simulink model "Modelo_Red_Mitigación_final"  (R2019b)
settings: Solver=VariableStepAuto  StartTime=0.0  StopTime=2.5  RelTol=1e-3
InitFcn:
  | Ts=20e-6;
undefined symbols (not defined in the file): D1, Delta, Ion, Lithium
libraries: powerlib x371, powerlib_meascontrol x286, simulink x50, simulink_extras x20, electricdrivelib x16
(part 8 of 11)

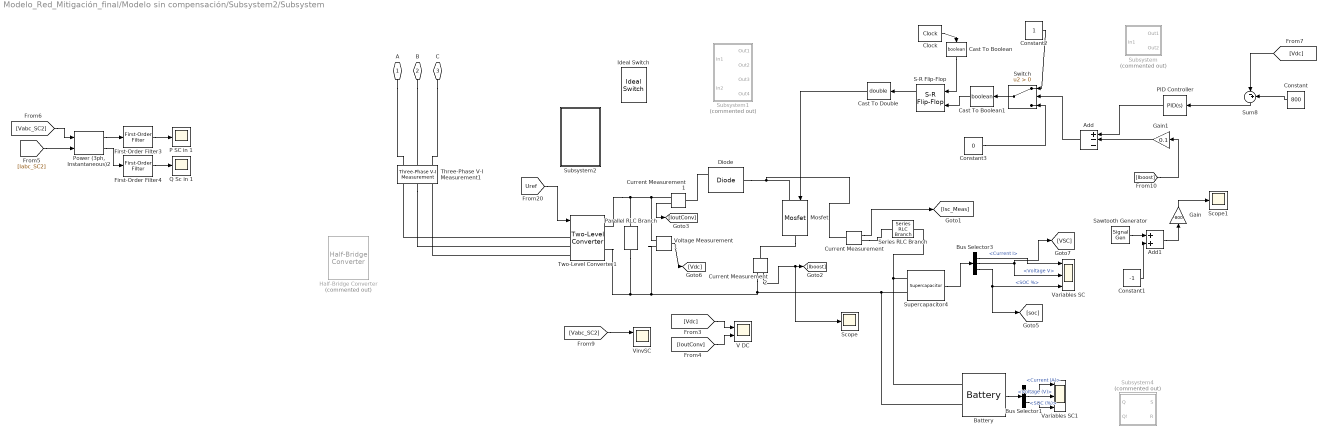
== system Modelo_Red_Mitigación_final/Modelo sin compensación/Subsystem2/Subsystem ==
  Add : Sum  Inputs=+--
  Add1 : Sum
  Battery : electricdrivelib/Extra Sources/Battery  BatType=Lithium-Ion  ShowTempParam=off  ThermalPreset=no  ShowAgeParam=off  NomV=500  NomQ=500  SOC=100  Batt_Tr=30  PresetModel=on  MaxQ=500  MinV=375  FullV=581.9936  Dis_rate=217.3913  R=0.01  Normal_OP=452.1739  expZone="[540.1929      24.56522]"  current=[6.5 13 32.5]  Units=Time  Tci=20  NomT=20  T2=-30  MaxQ2=4.8  FullV2=7.1  Normal_OP2=5.655  expZone2="[6.58           1]"  Rca=0.6  ti=2000  Dp=0  Neq0=0  Tsim=1e6  Ta1=25  Qeol=5.4*0.9  Reol=0.013333*1.2  Char_age=[2.3478, 3]  Dis_age=[2.3478, 10]  N1=1500  N2=10500  N3=1000  N4=1400  Ta2=45  N5=950
      settings: SourceProductName=Simscape Electrical
  Bus Selector1 : BusSelector  OutputSignals=Current (A),Voltage (V),SOC (%)
  Bus Selector3 : BusSelector  OutputSignals=Current I,Voltage V,SOC %
  Cast To Boolean : DataTypeConversion  OutDataTypeStr=boolean
  Cast To Boolean1 : DataTypeConversion  OutDataTypeStr=boolean
  Cast To Double : DataTypeConversion  OutDataTypeStr=double
  Clock : simulink_extras/Flip Flops/Clock  period=1/10e3
  Constant : Constant  Value=800
  Constant1 : Constant  Value=-1
  Constant2 : Constant
  Constant3 : Constant  Value=0
  Current Measurement : powerlib/Measurements/Current Measurement  PhasorSimulation=off  OutputType=Complex  PSBequivalent=0
      settings: SourceProductName=Simscape Electrical
  Current Measurement1 : powerlib/Measurements/Current Measurement  PhasorSimulation=off  OutputType=Complex  PSBequivalent=0
      settings: SourceProductName=Simscape Electrical
  Current Measurement2 : powerlib/Measurements/Current Measurement  PhasorSimulation=off  OutputType=Complex  PSBequivalent=0
      settings: SourceProductName=Simscape Electrical
  Diode : powerlib/Power Electronics/Diode  Ron=0.001  Lon=0  Vf=0.8  IC=0  UseSnubber=0  Rs=500  Cs=250e-9  Measurements=on
      settings: SourceProductName=Simscape Electrical
  First-Order Filter3 : powerlib_meascontrol/Filters/First-Order Filter  FilterType=Lowpass  Tc=10e-3  Ts=0  Initialize=on  Vac_Init=[0, 0, 60]  Vdc_Init=0  PlotResponse=off  FreqRange="[0,  200,  1]"
      settings: SourceProductName=Simscape Electrical
  First-Order Filter4 : powerlib_meascontrol/Filters/First-Order Filter  FilterType=Lowpass  Tc=10e-3  Ts=0  Initialize=on  Vac_Init=[0, 0, 60]  Vdc_Init=0  PlotResponse=off  FreqRange="[0,  200,  1]"
      settings: SourceProductName=Simscape Electrical
  Gain : Gain  Gain=-800
  Gain1 : Gain  Gain=0.1
  Half-Bridge Converter : powerlib/Power Electronics/Half-Bridge Converter  Commented=on  ModelType=Switching devices  Ron=1e-3  Rs=1e6  Cs=inf  Vforward=[0,0]  Ron_Diode=1e-3  Rs_Diode=1e6  Cs_Diode=inf  Vf_Diode=1e-3  Rs_CurrentSource=inf
      settings: SourceProductName=Simscape Electrical  SourceProductBaseCode=PS
  Ideal Switch : powerlib/Power Electronics/Ideal Switch  Ron=1e-3  Lon=0  IC=1  Rs=1e5  Cs=inf  Measurements=on
      settings: SourceProductName=Simscape Electrical
  Mosfet : powerlib/Power Electronics/Mosfet  Ron=0.1  Lon=0  Rd=0.01  Vfd=0  IC=0  Rs=1e5  Cs=inf  Measurements=off
      settings: SourceProductName=Simscape Electrical
  P SC in 1 : Scope
  PID Controller : simulink/Continuous/PID Controller  Controller=PID  Form=Parallel  TimeDomain=Continuous-time  SampleTime=-1  IntegratorMethod=Forward Euler  FilterMethod=Forward Euler  ControllerParametersSource=internal  P=40  I=10  D=0  UseFilter=on  N=100  TunerSelectOption=Transfer Function Based (PID Tuner App)  InitialConditionSource=internal  InitialConditionForIntegrator=0  InitialConditionForFilter=0  DifferentiatorICPrevScaledInput=0  ExternalReset=none  TrackingMode=off  Kt=1  LimitOutput=off  UpperSaturationLimit=inf  LowerSaturationLimit=-inf  LinearizeAsGain=on  AntiWindupMode=none  Kb=1  POutMin=[]  POutMax=[]  IOutMin=[]  IOutMax=[]  DOutMin=[]  DOutMax=[]  NOutMin=[]  NOutMax=[]  SumOutMin=[]  SumOutMax=[]  SaturationOutMin=[]  SaturationOutMax=[]  PParamMin=[]  PParamMax=[]  IParamMin=[]  IParamMax=[]  DParamMin=[]  DParamMax=[]  NParamMin=[]  NParamMax=[]  KbParamMin=[]  KbParamMax=[]  KtParamMin=[]  KtParamMax=[]  KbOutMin=[]  KbOutMax=[]  KtOutMin=[]  KtOutMax=[]  IntegratorOutMin=[]  IntegratorOutMax=[]  FilterOutMin=[]  FilterOutMax=[]  SumI1OutMin=[]  SumI1OutMax=[]  SumI2OutMin=[]  SumI2OutMax=[]  SumI3OutMin=[]  SumI3OutMax=[]  SumI4OutMin=[]  SumI4OutMax=[]  SumDOutMin=[]  SumDOutMax=[]  DifferentiatorOutMin=[]  DifferentiatorOutMax=[]  FilterDiffOutCoefMin=[]  FilterDiffOutCoefMax=[]  ReciprocalOutMin=[]  ReciprocalOutMax=[]  SumDenOutMin=[]  SumDenOutMax=[]  SumNumOutMin=[]  SumNumOutMax=[]  DivideOutMin=[]  DivideOutMax=[]  IntegratorContinuousStateAttributes=''  IntegratorStateMustResolveToSignalObject=off  IntegratorRTWStateStorageClass=Auto  FilterContinuousStateAttributes=''  FilterStateMustResolveToSignalObject=off  FilterRTWStateStorageClass=Auto  ParallelPVariant=InternalParameters  IdealPVariant=Disabled  IVariant=InternalParameters  DVariant=InternalParameters  IntegratorVariant=Continuous  SatVariant=Disabled  AWVariant=Passthrough  PCopyVariant=Disabled  TRVariant=Disabled  FdbkBlocksVariant=Forward  IdealPFdbkVariant=Disabled  SatFdbkVariant=Disabled  DerivativeFilterVariant=ContFilter  NVariant=InternalParameters  NCopyVariant=Disabled  FilterICVariant=InternalICsFilter  IntegratorICVariant=InternalICs  ExternalResetVariant=Disabled  TRSumVariant=Passthrough  SumFdbkVariant=Disabled  SumVariant=Sum_PID
  Parallel RLC Branch : powerlib/Elements/Parallel RLC Branch  LConnTagsString=a  RConnTagsString=__new0  BranchType=C  Resistance=0.01  Inductance=1e-3  SetiL0=off  InitialCurrent=0  Capacitance=6600e-6  Setx0=off  InitialVoltage=800  Measurements=None
      settings: SourceProductName=Simscape Electrical
  "Power (3ph, Instantaneous)2" : powerlib_meascontrol/Measurements/Power (3ph, Instantaneous)
      settings: SourceProductName=Simscape Electrical
  Q Sc in 1 : Scope
  S-R Flip-Flop : simulink_extras/Flip Flops/S-R Flip-Flop  initial_condition=1
  Sawtooth Generator : SignalGenerator  WaveForm=sawtooth  Frequency=10e3
  Scope : Scope
  Scope1 : Scope
  Series RLC Branch : powerlib/Elements/Series RLC Branch  LConnTagsString=__new0  RConnTagsString=__new0  BranchType=L  Resistance=65e-3  Inductance=1e-3  SetiL0=off  InitialCurrent=0  Capacitance=1e-6  Setx0=off  InitialVoltage=0  Measurements=None
      settings: SourceProductName=Simscape Electrical
  Subsystem : Subsystem  Commented=on
  Subsystem1 : Subsystem  Commented=on
  Subsystem2 : Subsystem
  Subsystem4 : Subsystem  Commented=on
  Sum8 : Sum  Inputs=|-+
  Supercapacitor4 : electricdrivelib/Extra Sources/Supercapacitor  C=18  Rdc=7e-3  Voltage=500  Ns=1  Np=1  Vinit=500  Temp=25  PresetModel=on  EstParam=off  Nc=1  r=1e-9  epsilon=6.0208e-10  Ich=10  Vstern="[0.161  2.7  7.8]"  Self_dis=off  Ioc=10  Vself="[48  47.8  47.06  44.65]"  demandeplot=off  I="[10  20 100  500]"  Units=sec  Vmax=0  If=0  deltaV=0  alpha=0  sec=0
      settings: SourceProductName=Simscape Electrical  SourceProductBaseCode=PS
  Switch : Switch  Criteria=u2 > Threshold
  Three-Phase V-I Measurement1 : powerlib/Measurements/Three-Phase V-I Measurement  VoltageMeasurement=phase-to-phase  SetLabelV=on  LabelV=Vabc_SC2  Vpu=off  VpuLL=off  CurrentMeasurement=yes  SetLabelI=on  LabelI=Iabc_SC2  Ipu=off  Pbase=100e6  Vbase=500e3  OutputType=Complex  PhasorSimulation=off  PSBequivalent=0
      settings: SourceProductName=Simscape Electrical
  Two-Level Converter1 : powerlib/Power Electronics/Two-Level Converter  ModelType=Average model (Uref-controlled)  Ron=1e-3  Rs=1e6  Cs=inf  Vforward=[0,0]  Ron_Diode=1e-3  Rs_Diode=1e6  Cs_Diode=inf  Vf_Diode=1e-3  Rs_CurrentSource=inf
      settings: SourceProductName=Simscape Electrical  SourceProductBaseCode=PS
  V DC : Scope  NumInputPorts=2
  Variables SC : Scope  NumInputPorts=3
  Variables SC1 : Scope  NumInputPorts=3
  VinvSC : Scope  NumInputPorts=2
  Voltage Measurement1 : powerlib/Measurements/Voltage Measurement  PhasorSimulation=off  OutputType=Complex  PSBequivalent=0
      settings: SourceProductName=Simscape Electrical
  A : PMIOPort  Side=Left
  B : PMIOPort  Port=2  Side=Left
  C : PMIOPort  Port=3  Side=Left
  wires:
  Current Measurement/1 -> [Isc_Meas]
  Bus Selector3/2 -> Variables SC/2, [VSC]  "<Voltage V>"
  Bus Selector3/3 -> [soc], Variables SC/3  "<SOC %>"
  Bus Selector3/1 -> Variables SC/1  "<Current I>"
  "Power (3ph, Instantaneous)2"/2 -> First-Order Filter4/1
  [Iabc_SC2] -> "Power (3ph, Instantaneous)2"/2
  First-Order Filter3/1 -> P SC in 1/1
  [Vabc_SC2] -> "Power (3ph, Instantaneous)2"/1
  First-Order Filter4/1 -> Q Sc in 1/1
  "Power (3ph, Instantaneous)2"/1 -> First-Order Filter3/1
  [Vabc_SC2] -> VinvSC/1
  Voltage Measurement1/1 -> [Vdc]
  [Uref] -> Two-Level Converter1/1
  Current Measurement1/1 -> [IoutConv]
  [Vdc] -> V DC/1
  [IoutConv] -> V DC/2
  Supercapacitor4/1 -> Bus Selector3/1
  Current Measurement2/1 -> Scope/1, [Iboost]
  [Iboost] -> Gain1/1
  Constant/1 -> Sum8/2
  [Vdc] -> Sum8/1
  Cast To Boolean1/1 -> S-R Flip-Flop/2
  Cast To Double/1 -> Mosfet/1
  Clock/1 -> Cast To Boolean/1
  Add/1 -> Switch/2
  Cast To Boolean/1 -> S-R Flip-Flop/1
  S-R Flip-Flop/1 -> Cast To Double/1
  Constant3/1 -> Switch/3
  Switch/1 -> Cast To Boolean1/1
  Constant2/1 -> Switch/1
  Sum8/1 -> PID Controller/1
  Bus Selector1/2 -> Variables SC1/2  "<Voltage (V)>"
  Battery/1 -> Bus Selector1/1
  Bus Selector1/3 -> Variables SC1/3  "<SOC (%)>"
  Bus Selector1/1 -> Variables SC1/1  "<Current (A)>"
  Gain1/1 -> Add/2
  PID Controller/1 -> Add/1
  Sawtooth Generator/1 -> Add1/1
  Add1/1 -> Gain/1
  Constant1/1 -> Add1/2
  Gain/1 -> Scope1/1
  connections:
  Current Measurement/RConn1 -- Series RLC Branch/LConn1
  Voltage Measurement1/LConn2 -- Battery/LConn2 -- Supercapacitor4/LConn2 -- Current Measurement2/RConn1 -- Two-Level Converter1/RConn2 -- Parallel RLC Branch/RConn1
  B/RConn1 -- Three-Phase V-I Measurement1/LConn2
  C/RConn1 -- Three-Phase V-I Measurement1/LConn3
  A/RConn1 -- Three-Phase V-I Measurement1/LConn1
  Parallel RLC Branch/LConn1 -- Two-Level Converter1/RConn1 -- Current Measurement1/RConn1 -- Voltage Measurement1/LConn1
  Diode/LConn1 -- Mosfet/LConn1 -- Current Measurement/LConn1
  Two-Level Converter1/LConn1 -- Three-Phase V-I Measurement1/RConn1
  Three-Phase V-I Measurement1/RConn2 -- Two-Level Converter1/LConn2
  Two-Level Converter1/LConn3 -- Three-Phase V-I Measurement1/RConn3
  Mosfet/RConn1 -- Current Measurement2/LConn1
  Diode/RConn1 -- Current Measurement1/LConn1
  Supercapacitor4/LConn1 -- Battery/LConn1 -- Series RLC Branch/RConn1

== system Modelo_Red_Mitigación_final/Modelo SC pasivo/Subsystem2/Subsystem/Subsystem ==
  In1 : Inport
  Cast To Boolean : DataTypeConversion  OutDataTypeStr=boolean
  Cast To Boolean1 : DataTypeConversion  OutDataTypeStr=boolean
  Cast To Double : DataTypeConversion  OutDataTypeStr=double
  Clock : simulink_extras/Flip Flops/Clock  period=1/10e3
  Constant1 : Constant  Value=0
  Constant2 : Constant
  Constant3 : Constant  Value=0
  Mux : Mux  Inputs=2
  S-R Flip-Flop : simulink_extras/Flip Flops/S-R Flip-Flop  initial_condition=1
  Switch : Switch  Criteria=u2 > Threshold
  Out1 : Outport
  Out2 : Outport  Port=2
  wires:
  S-R Flip-Flop/1 -> Cast To Double/1
  Constant2/1 -> Switch/1
  Cast To Double/1 -> Mux/2
  Cast To Boolean/1 -> S-R Flip-Flop/1
  Constant1/1 -> Mux/1
  Constant3/1 -> Switch/3
  Switch/1 -> Cast To Boolean1/1
  Cast To Boolean1/1 -> S-R Flip-Flop/2
  Mux/1 -> Out1/1
  Clock/1 -> Cast To Boolean/1
  In1/1 -> Switch/2
  S-R Flip-Flop/2 -> Out2/1

== system Modelo_Red_Mitigación_final/Modelo SC pasivo/Subsystem2/Subsystem/Subsystem1 ==
  In1 : Inport
  In2 : Inport  Port=2
  Constant2 : Constant
  Constant3 : Constant  Value=100
  Constant4 : Constant
  Demux1 : Demux  Outputs=3
  First-Order Filter : powerlib_meascontrol/Filters/First-Order Filter  FilterType=Lowpass  Tc=10e-3  Ts=0  Initialize=on  Vac_Init=[0, 0, 60]  Vdc_Init=0  PlotResponse=off  FreqRange="[0,  200,  1]"
      settings: SourceProductName=Simscape Electrical
  Gain : Gain  Gain=1/1200
  Gain1 : Gain  Gain=pi/180
  Gain2 : Gain  Gain=1/254
  Gain3 : Gain  Gain=1/30e3
  Isc : Scope
  MATLAB Function : MATLAB Function  TreatAsAtomicUnit=on
  Memory1 : Memory
  Memory2 : Memory
  Mux2 : Mux  Inputs=3
  Mux3 : Mux  Inputs=3
  PID Controller1 : simulink/Continuous/PID Controller  Controller=PID  Form=Parallel  TimeDomain=Discrete-time  SampleTime=-1  IntegratorMethod=Forward Euler  FilterMethod=Forward Euler  ControllerParametersSource=internal  P=0.4  I=1  D=0  UseFilter=off  N=100  TunerSelectOption=Transfer Function Based (PID Tuner App)  InitialConditionSource=internal  InitialConditionForIntegrator=0.5  InitialConditionForFilter=0.5  DifferentiatorICPrevScaledInput=0  ExternalReset=none  TrackingMode=off  Kt=1  LimitOutput=off  UpperSaturationLimit=inf  LowerSaturationLimit=-inf  LinearizeAsGain=on  AntiWindupMode=none  Kb=1  POutMin=[]  POutMax=[]  IOutMin=[]  IOutMax=[]  DOutMin=[]  DOutMax=[]  NOutMin=[]  NOutMax=[]  SumOutMin=[]  SumOutMax=[]  SaturationOutMin=[]  SaturationOutMax=[]  PParamMin=[]  PParamMax=[]  IParamMin=[]  IParamMax=[]  DParamMin=[]  DParamMax=[]  NParamMin=[]  NParamMax=[]  KbParamMin=[]  KbParamMax=[]  KtParamMin=[]  KtParamMax=[]  KbOutMin=[]  KbOutMax=[]  KtOutMin=[]  KtOutMax=[]  IntegratorOutMin=[]  IntegratorOutMax=[]  FilterOutMin=[]  FilterOutMax=[]  SumI1OutMin=[]  SumI1OutMax=[]  SumI2OutMin=[]  SumI2OutMax=[]  SumI3OutMin=[]  SumI3OutMax=[]  SumI4OutMin=[]  SumI4OutMax=[]  SumDOutMin=[]  SumDOutMax=[]  DifferentiatorOutMin=[]  DifferentiatorOutMax=[]  FilterDiffOutCoefMin=[]  FilterDiffOutCoefMax=[]  ReciprocalOutMin=[]  ReciprocalOutMax=[]  SumDenOutMin=[]  SumDenOutMax=[]  SumNumOutMin=[]  SumNumOutMax=[]  DivideOutMin=[]  DivideOutMax=[]  IntegratorContinuousStateAttributes=''  IntegratorStateMustResolveToSignalObject=off  IntegratorRTWStateStorageClass=Auto  FilterContinuousStateAttributes=''  FilterStateMustResolveToSignalObject=off  FilterRTWStateStorageClass=Auto  ParallelPVariant=InternalParameters  IdealPVariant=Disabled  IVariant=InternalParameters  DVariant=InternalParameters  IntegratorVariant=Discrete  SatVariant=Disabled  AWVariant=Passthrough  PCopyVariant=Disabled  TRVariant=Disabled  FdbkBlocksVariant=Forward  IdealPFdbkVariant=Disabled  SatFdbkVariant=Disabled  DerivativeFilterVariant=Differentiator  NVariant=Passthrough  NCopyVariant=Disabled_SignalSpec  FilterICVariant=InternalICsDifferentiator  IntegratorICVariant=InternalICs  ExternalResetVariant=Disabled  TRSumVariant=Passthrough  SumFdbkVariant=Disabled  SumVariant=Sum_PID
  PID Controller4 : simulink/Continuous/PID Controller  Controller=PID  Form=Parallel  TimeDomain=Discrete-time  SampleTime=-1  IntegratorMethod=Forward Euler  FilterMethod=Forward Euler  ControllerParametersSource=internal  P=0.001  I=0.06  D=0  UseFilter=off  N=100  TunerSelectOption=Transfer Function Based (PID Tuner App)  InitialConditionSource=internal  InitialConditionForIntegrator=0.5  InitialConditionForFilter=0.5  DifferentiatorICPrevScaledInput=0  ExternalReset=none  TrackingMode=off  Kt=1  LimitOutput=off  UpperSaturationLimit=inf  LowerSaturationLimit=-inf  LinearizeAsGain=on  AntiWindupMode=none  Kb=1  POutMin=[]  POutMax=[]  IOutMin=[]  IOutMax=[]  DOutMin=[]  DOutMax=[]  NOutMin=[]  NOutMax=[]  SumOutMin=[]  SumOutMax=[]  SaturationOutMin=[]  SaturationOutMax=[]  PParamMin=[]  PParamMax=[]  IParamMin=[]  IParamMax=[]  DParamMin=[]  DParamMax=[]  NParamMin=[]  NParamMax=[]  KbParamMin=[]  KbParamMax=[]  KtParamMin=[]  KtParamMax=[]  KbOutMin=[]  KbOutMax=[]  KtOutMin=[]  KtOutMax=[]  IntegratorOutMin=[]  IntegratorOutMax=[]  FilterOutMin=[]  FilterOutMax=[]  SumI1OutMin=[]  SumI1OutMax=[]  SumI2OutMin=[]  SumI2OutMax=[]  SumI3OutMin=[]  SumI3OutMax=[]  SumI4OutMin=[]  SumI4OutMax=[]  SumDOutMin=[]  SumDOutMax=[]  DifferentiatorOutMin=[]  DifferentiatorOutMax=[]  FilterDiffOutCoefMin=[]  FilterDiffOutCoefMax=[]  ReciprocalOutMin=[]  ReciprocalOutMax=[]  SumDenOutMin=[]  SumDenOutMax=[]  SumNumOutMin=[]  SumNumOutMax=[]  DivideOutMin=[]  DivideOutMax=[]  IntegratorContinuousStateAttributes=''  IntegratorStateMustResolveToSignalObject=off  IntegratorRTWStateStorageClass=Auto  FilterContinuousStateAttributes=''  FilterStateMustResolveToSignalObject=off  FilterRTWStateStorageClass=Auto  ParallelPVariant=InternalParameters  IdealPVariant=Disabled  IVariant=InternalParameters  DVariant=InternalParameters  IntegratorVariant=Discrete  SatVariant=Disabled  AWVariant=Passthrough  PCopyVariant=Disabled  TRVariant=Disabled  FdbkBlocksVariant=Forward  IdealPFdbkVariant=Disabled  SatFdbkVariant=Disabled  DerivativeFilterVariant=Differentiator  NVariant=Passthrough  NCopyVariant=Disabled_SignalSpec  FilterICVariant=InternalICsDifferentiator  IntegratorICVariant=InternalICs  ExternalResetVariant=Disabled  TRSumVariant=Passthrough  SumFdbkVariant=Disabled  SumVariant=Sum_PID
  PLL (3ph)1 : powerlib_meascontrol/PLL/PLL (3ph)  Fmin=45  Par_Init=[0, 60]  ParK=[180, 3200, 1]  TcD=1e-4  MaxRateChangeFreq=12  FilterCutOffFreq=25  Ts=0  AGC=on
      settings: SourceProductName=Simscape Electrical
  "Power (3ph, Instantaneous)" : powerlib_meascontrol/Measurements/Power (3ph, Instantaneous)
      settings: SourceProductName=Simscape Electrical
  Product : Product
  Product1 : Product
  RMS16 : powerlib_meascontrol/Measurements/RMS  TrueRMS=on  Freq=60  RMSInit=19.9e3  Ts=0
      settings: SourceProductName=Simscape Electrical
  Sin : Trigonometry
  Sum1 : Sum  Inputs=|-+
  Sum4 : Sum  Inputs=+-|
  Sum5 : Sum  Inputs=-+|
  Switch2 : Switch  Criteria=u2 > Threshold  Threshold=0.9
  Tensión bus DC1 : Scope
  Transport Delay : TransportDelay  DelayTime=11.06e-3
  Transport Delay1 : TransportDelay  DelayTime=5.53e-3
  Transport Delay2 : TransportDelay  DelayTime=11.06e-3
  Transport Delay3 : TransportDelay  DelayTime=5.53e-3
  "Uccm " : Scope
  "Uvcm " : Scope
  Out1 : Outport
  Out2 : Outport  Port=2
  Out3 : Outport  Port=3
  Out4 : Outport  Port=4
  wires:
  Gain2/1 -> MATLAB Function/1(u), Switch2/2
  Product1/1 -> Mux3/1, Transport Delay2/1, Transport Delay3/1
  Sin/1 -> [Vabc_sync], Product/1
  [VCli1BT] -> "Power (3ph, Instantaneous)"/1  "V_C2"
  Transport Delay/1 -> Mux2/3
  In2/1 -> [VoutConv]
  Sum5/1 -> Sin/1
  PLL (3ph)1/1 -> Out4/1
  Mux2/1 -> Switch2/1, "Uvcm "/1
  "Power (3ph, Instantaneous)"/1 -> First-Order Filter/1
  Gain/1 -> PID Controller1/1
  Transport Delay2/1 -> Mux3/3
  [soc] -> MATLAB Function/2(soc)
  Product/1 -> Mux2/1, Transport Delay1/1, Transport Delay/1
  Constant4/1 -> Product/2
  PLL (3ph)1/2 -> Sum5/2
  Mux3/1 -> Switch2/3, "Uccm "/1
  [Vabc_sync] -> Product1/1
  [VCli1BT] -> Memory2/1
  Constant2/1 -> Product1/2
  First-Order Filter/1 -> Gain3/1
  MATLAB Function/1(y) -> [Isc_Ref], Isc/1
  Transport Delay1/1 -> Mux2/2
  RMS16/1 -> Gain2/1
  Transport Delay3/1 -> Mux3/2
  "Power (3ph, Instantaneous)"/2 -> Out3/1
  PID Controller4/1 -> Gain1/1
  Memory2/1 -> PLL (3ph)1/1
  Gain3/1 -> Sum4/2
  Demux1/1 -> RMS16/1
  Constant3/1 -> Sum1/2
  PID Controller1/1 -> Tensión bus DC1/1, Sum4/1
  Demux1/3 -> Out2/1
  Gain1/1 -> Sum5/1
  [VCli1BT_1] -> Demux1/1
  In1/1 -> Sum1/1
  Memory1/1 -> PID Controller4/1
  Sum4/1 -> Memory1/1
  Demux1/2 -> Out1/1
  Switch2/1 -> [Uref]
  [ICli1BT] -> "Power (3ph, Instantaneous)"/2  "I_SC Red"
  Sum1/1 -> Gain/1

== system Modelo_Red_Mitigación_final/Modelo SC pasivo/Subsystem2/Subsystem/Subsystem2 ==
  Add : Sum  Inputs=-+
  Constant : Constant  Value=0.95
  Constant1 : Constant  Value=0
  Discrete PID Controller : simulink/Continuous/PID Controller  Controller=PID  Form=Parallel  TimeDomain=Discrete-time  SampleTime=-1  IntegratorMethod=Forward Euler  FilterMethod=Forward Euler  ControllerParametersSource=internal  P=20  I=2  D=0  UseFilter=off  N=100  TunerSelectOption=Transfer Function Based (PID Tuner App)  InitialConditionSource=internal  InitialConditionForIntegrator=0  InitialConditionForFilter=0  DifferentiatorICPrevScaledInput=0  ExternalReset=none  TrackingMode=off  Kt=1  LimitOutput=off  UpperSaturationLimit=inf  LowerSaturationLimit=-inf  LinearizeAsGain=off  AntiWindupMode=none  Kb=1  POutMin=[]  POutMax=[]  IOutMin=[]  IOutMax=[]  DOutMin=[]  DOutMax=[]  NOutMin=[]  NOutMax=[]  SumOutMin=[]  SumOutMax=[]  SaturationOutMin=[]  SaturationOutMax=[]  PParamMin=[]  PParamMax=[]  IParamMin=[]  IParamMax=[]  DParamMin=[]  DParamMax=[]  NParamMin=[]  NParamMax=[]  KbParamMin=[]  KbParamMax=[]  KtParamMin=[]  KtParamMax=[]  KbOutMin=[]  KbOutMax=[]  KtOutMin=[]  KtOutMax=[]  IntegratorOutMin=[]  IntegratorOutMax=[]  FilterOutMin=[]  FilterOutMax=[]  SumI1OutMin=[]  SumI1OutMax=[]  SumI2OutMin=[]  SumI2OutMax=[]  SumI3OutMin=[]  SumI3OutMax=[]  SumI4OutMin=[]  SumI4OutMax=[]  SumDOutMin=[]  SumDOutMax=[]  DifferentiatorOutMin=[]  DifferentiatorOutMax=[]  FilterDiffOutCoefMin=[]  FilterDiffOutCoefMax=[]  ReciprocalOutMin=[]  ReciprocalOutMax=[]  SumDenOutMin=[]  SumDenOutMax=[]  SumNumOutMin=[]  SumNumOutMax=[]  DivideOutMin=[]  DivideOutMax=[]  IntegratorContinuousStateAttributes=''  IntegratorStateMustResolveToSignalObject=off  IntegratorRTWStateStorageClass=Auto  FilterContinuousStateAttributes=''  FilterStateMustResolveToSignalObject=off  FilterRTWStateStorageClass=Auto  ParallelPVariant=InternalParameters  IdealPVariant=Disabled  IVariant=InternalParameters  DVariant=InternalParameters  IntegratorVariant=Discrete  SatVariant=Disabled  AWVariant=Passthrough  PCopyVariant=Disabled  TRVariant=Disabled  FdbkBlocksVariant=Forward  IdealPFdbkVariant=Disabled  SatFdbkVariant=Disabled  DerivativeFilterVariant=Differentiator  NVariant=Passthrough  NCopyVariant=Disabled_SignalSpec  FilterICVariant=InternalICsDifferentiator  IntegratorICVariant=InternalICs  ExternalResetVariant=Disabled  TRSumVariant=Passthrough  SumFdbkVariant=Disabled  SumVariant=Sum_PID
  First-Order Filter : powerlib_meascontrol/Filters/First-Order Filter  FilterType=Lowpass  Tc=1e-3  Ts=0  Initialize=off  Vac_Init=[0, 0, 60]  Vdc_Init=0  PlotResponse=off  FreqRange="[0,  200,  1]"
      settings: SourceProductName=Simscape Electrical
  Gain : Gain  Gain=1/(254*sqrt(2))
  Mux : Mux  Inputs=2
  Mux1 : Mux  Inputs=2
  PLL (3ph) : powerlib_meascontrol/PLL/PLL (3ph)  Fmin=45  Par_Init=[0, 60]  ParK=[180, 3200, 1]  TcD=1e-4  MaxRateChangeFreq=12  FilterCutOffFreq=25  Ts=0  AGC=on
      settings: SourceProductName=Simscape Electrical
  Selector : Selector  InputPortWidth=3  IndexOptions=Index vector (dialog)  Indices=[1 2]  OutputSizes=1
  abc to dq0 : powerlib_meascontrol/Transformations/abc to dq0  Alignment=90 degrees behind phase A axis
      settings: SourceProductName=Simscape Electrical
  dq0 to abc : powerlib_meascontrol/Transformations/dq0 to abc  Alignment=90 degrees behind phase A axis
      settings: SourceProductName=Simscape Electrical
  tag scope: Uref=global
  wires:
  [VCli1BT] -> PLL (3ph)/1
  abc to dq0/1 -> Gain/1
  Selector/1 -> Add/1
  Mux/1 -> Add/2
  [wt] -> dq0 to abc/2
  dq0 to abc/1 -> [Uref]
  [VCli1BT_1] -> First-Order Filter/1
  Discrete PID Controller/1 -> Mux1/1
  Mux1/1 -> dq0 to abc/1
  Add/1 -> Discrete PID Controller/1
  First-Order Filter/1 -> abc to dq0/1
  Gain/1 -> Selector/1
  PLL (3ph)/2 -> [wt], abc to dq0/2
  Constant/1 -> Mux/1
  Constant1/1 -> Mux/2, Mux1/2

== system Modelo_Red_Mitigación_final/Modelo SC pasivo/Subsystem2/Subsystem/Subsystem4 ==
  S : Inport
  R : Inport  Port=2
  Combinatorial Logic : CombinatorialLogic  TruthTable=[0 1;1 0;0 1;1 1;1 0;1 0;0 0;1 1]
  Demux : Demux  Outputs=2
  Memory : Memory  InitialCondition=1
  Mux : Mux  Inputs=3
  Q : Outport
  Q! : Outport  Port=2
  wires:
  Mux/1 -> Combinatorial Logic/1
  Demux/1 -> Q/1, Memory/1
  Combinatorial Logic/1 -> Demux/1
  Demux/2 -> Q!/1
  S/1 -> Mux/1
  Memory/1 -> Mux/3
  R/1 -> Mux/2

== system Modelo_Red_Mitigación_final/Modelo SC pasivo/Subsystem3/Subsystem2/AC_CONTROL ALGORITHM ==
  Add : Sum  Inputs=-+
  Constant : Constant  Value=1.1
  Constant1 : Constant  Value=0
  Constant2 : Constant  Value=0
  Constant3 : Constant
  Demux1 : Demux  Outputs=3
  Discrete PID Controller : simulink/Continuous/PID Controller  Controller=PID  Form=Parallel  TimeDomain=Continuous-time  SampleTime=-1  IntegratorMethod=Forward Euler  FilterMethod=Forward Euler  ControllerParametersSource=internal  P=5  I=1  D=0  UseFilter=on  N=100  TunerSelectOption=Transfer Function Based (PID Tuner App)  InitialConditionSource=internal  InitialConditionForIntegrator=0  InitialConditionForFilter=0  DifferentiatorICPrevScaledInput=0  ExternalReset=none  TrackingMode=off  Kt=1  LimitOutput=off  UpperSaturationLimit=inf  LowerSaturationLimit=-inf  LinearizeAsGain=off  AntiWindupMode=none  Kb=1  POutMin=[]  POutMax=[]  IOutMin=[]  IOutMax=[]  DOutMin=[]  DOutMax=[]  NOutMin=[]  NOutMax=[]  SumOutMin=[]  SumOutMax=[]  SaturationOutMin=[]  SaturationOutMax=[]  PParamMin=[]  PParamMax=[]  IParamMin=[]  IParamMax=[]  DParamMin=[]  DParamMax=[]  NParamMin=[]  NParamMax=[]  KbParamMin=[]  KbParamMax=[]  KtParamMin=[]  KtParamMax=[]  KbOutMin=[]  KbOutMax=[]  KtOutMin=[]  KtOutMax=[]  IntegratorOutMin=[]  IntegratorOutMax=[]  FilterOutMin=[]  FilterOutMax=[]  SumI1OutMin=[]  SumI1OutMax=[]  SumI2OutMin=[]  SumI2OutMax=[]  SumI3OutMin=[]  SumI3OutMax=[]  SumI4OutMin=[]  SumI4OutMax=[]  SumDOutMin=[]  SumDOutMax=[]  DifferentiatorOutMin=[]  DifferentiatorOutMax=[]  FilterDiffOutCoefMin=[]  FilterDiffOutCoefMax=[]  ReciprocalOutMin=[]  ReciprocalOutMax=[]  SumDenOutMin=[]  SumDenOutMax=[]  SumNumOutMin=[]  SumNumOutMax=[]  DivideOutMin=[]  DivideOutMax=[]  IntegratorContinuousStateAttributes=''  IntegratorStateMustResolveToSignalObject=off  IntegratorRTWStateStorageClass=Auto  FilterContinuousStateAttributes=''  FilterStateMustResolveToSignalObject=off  FilterRTWStateStorageClass=Auto  ParallelPVariant=InternalParameters  IdealPVariant=Disabled  IVariant=InternalParameters  DVariant=InternalParameters  IntegratorVariant=Continuous  SatVariant=Disabled  AWVariant=Passthrough  PCopyVariant=Disabled  TRVariant=Disabled  FdbkBlocksVariant=Forward  IdealPFdbkVariant=Disabled  SatFdbkVariant=Disabled  DerivativeFilterVariant=ContFilter  NVariant=InternalParameters  NCopyVariant=Disabled  FilterICVariant=InternalICsFilter  IntegratorICVariant=InternalICs  ExternalResetVariant=Disabled  TRSumVariant=Passthrough  SumFdbkVariant=Disabled  SumVariant=Sum_PID
  First-Order Filter : powerlib_meascontrol/Filters/First-Order Filter  FilterType=Lowpass  Tc=1e-3  Ts=0  Initialize=off  Vac_Init=[0, 0, 60]  Vdc_Init=0  PlotResponse=off  FreqRange="[0,  200,  1]"
      settings: SourceProductName=Simscape Electrical
  Gain : Gain  Gain=1/(19900*sqrt(2)*0.95)
  Limiting max Voltage : Saturate  UpperLimit=1  LowerLimit=-1
  Mux : Mux  Inputs=2
  Mux1 : Mux  Inputs=2
  PLL (3ph) : powerlib_meascontrol/PLL/PLL (3ph)  Fmin=45  Par_Init=[0, 60]  ParK=[180, 3200, 1]  TcD=1e-4  MaxRateChangeFreq=12  FilterCutOffFreq=25  Ts=0  AGC=on
      settings: SourceProductName=Simscape Electrical
  RMS : powerlib_meascontrol/Measurements/RMS  TrueRMS=on  Freq=60  RMSInit=18100  Ts=0
      settings: SourceProductName=Simscape Electrical
  Selector : Selector  InputPortWidth=3  IndexOptions=Index vector (dialog)  Indices=[1 2]  OutputSizes=1
  Switch : Switch  Criteria=u2 > Threshold  Threshold=18000
  Terminator2 : Terminator
  Terminator3 : Terminator
  abc to dq0 : powerlib_meascontrol/Transformations/abc to dq0  Alignment=90 degrees behind phase A axis
      settings: SourceProductName=Simscape Electrical
  dq0 to abc : powerlib_meascontrol/Transformations/dq0 to abc  Alignment=90 degrees behind phase A axis
      settings: SourceProductName=Simscape Electrical
  tag scope: Uref=global
  wires:
  [VCli1BT2] -> Demux1/1, PLL (3ph)/1
  abc to dq0/1 -> Gain/1
  Selector/1 -> Add/1
  Mux/1 -> Add/2
  [wt] -> dq0 to abc/2
  dq0 to abc/1 -> [Uref]
  [VCli1BT_2] -> First-Order Filter/1
  Mux1/1 -> dq0 to abc/1
  Add/1 -> Discrete PID Controller/1
  First-Order Filter/1 -> abc to dq0/1
  Gain/1 -> Selector/1
  PLL (3ph)/2 -> [wt], abc to dq0/2
  Discrete PID Controller/1 -> Limiting max Voltage/1
  Limiting max Voltage/1 -> Mux1/1
  Constant1/1 -> Mux1/2
  Constant2/1 -> Mux/2
  Constant3/1 -> Switch/1
  Constant/1 -> Switch/3
  Switch/1 -> Mux/1
  Demux1/1 -> RMS/1
  RMS/1 -> Switch/2
  Demux1/2 -> Terminator2/1
  Demux1/3 -> Terminator3/1

== system Modelo_Red_Mitigación_final/Modelo SC pasivo/Subsystem3/Subsystem2/Control1 ==
  Add1 : Sum  Inputs=+-
  Add3 : Sum  Inputs=+-
  Cast To Double : DataTypeConversion  OutDataTypeStr=double
  Constant : Constant  Value=1500
  Gain : Gain  Gain=1500/1000
  Mux : Mux  Inputs=2
  NOT : Logic  Operator=NOT  IconShape=distinctive  AllPortsSameDT=off  OutDataTypeStr=boolean
  PID Controller : simulink/Continuous/PID Controller  Controller=PID  Form=Parallel  TimeDomain=Continuous-time  SampleTime=-1  IntegratorMethod=Forward Euler  FilterMethod=Forward Euler  ControllerParametersSource=internal  P=0.4  I=0.4  D=0  UseFilter=on  N=100  TunerSelectOption=Transfer Function Based (PID Tuner App)  InitialConditionSource=internal  InitialConditionForIntegrator=0  InitialConditionForFilter=0  DifferentiatorICPrevScaledInput=0  ExternalReset=none  TrackingMode=off  Kt=1  LimitOutput=off  UpperSaturationLimit=250  LowerSaturationLimit=-250  LinearizeAsGain=on  AntiWindupMode=back-calculation  Kb=1  POutMin=[]  POutMax=[]  IOutMin=[]  IOutMax=[]  DOutMin=[]  DOutMax=[]  NOutMin=[]  NOutMax=[]  SumOutMin=[]  SumOutMax=[]  SaturationOutMin=[]  SaturationOutMax=[]  PParamMin=[]  PParamMax=[]  IParamMin=[]  IParamMax=[]  DParamMin=[]  DParamMax=[]  NParamMin=[]  NParamMax=[]  KbParamMin=[]  KbParamMax=[]  KtParamMin=[]  KtParamMax=[]  KbOutMin=[]  KbOutMax=[]  KtOutMin=[]  KtOutMax=[]  IntegratorOutMin=[]  IntegratorOutMax=[]  FilterOutMin=[]  FilterOutMax=[]  SumI1OutMin=[]  SumI1OutMax=[]  SumI2OutMin=[]  SumI2OutMax=[]  SumI3OutMin=[]  SumI3OutMax=[]  SumI4OutMin=[]  SumI4OutMax=[]  SumDOutMin=[]  SumDOutMax=[]  DifferentiatorOutMin=[]  DifferentiatorOutMax=[]  FilterDiffOutCoefMin=[]  FilterDiffOutCoefMax=[]  ReciprocalOutMin=[]  ReciprocalOutMax=[]  SumDenOutMin=[]  SumDenOutMax=[]  SumNumOutMin=[]  SumNumOutMax=[]  DivideOutMin=[]  DivideOutMax=[]  IntegratorContinuousStateAttributes=''  IntegratorStateMustResolveToSignalObject=off  IntegratorRTWStateStorageClass=Auto  FilterContinuousStateAttributes=''  FilterStateMustResolveToSignalObject=off  FilterRTWStateStorageClass=Auto  ParallelPVariant=InternalParameters  IdealPVariant=Disabled  IVariant=InternalParameters  DVariant=InternalParameters  IntegratorVariant=Continuous  SatVariant=Disabled  AWVariant=Passthrough  PCopyVariant=Disabled  TRVariant=Disabled  FdbkBlocksVariant=Forward  IdealPFdbkVariant=Disabled  SatFdbkVariant=Disabled  DerivativeFilterVariant=ContFilter  NVariant=InternalParameters  NCopyVariant=Disabled  FilterICVariant=InternalICsFilter  IntegratorICVariant=InternalICs  ExternalResetVariant=Disabled  TRSumVariant=Passthrough  SumFdbkVariant=Disabled  SumVariant=Sum_PID
  PID Controller1 : simulink/Continuous/PID Controller  Controller=PID  Form=Parallel  TimeDomain=Discrete-time  SampleTime=-1  IntegratorMethod=Forward Euler  FilterMethod=Forward Euler  ControllerParametersSource=internal  P=0.5  I=0.2  D=0  UseFilter=on  N=100  TunerSelectOption=Transfer Function Based (PID Tuner App)  InitialConditionSource=internal  InitialConditionForIntegrator=0  InitialConditionForFilter=0  DifferentiatorICPrevScaledInput=0  ExternalReset=none  TrackingMode=off  Kt=1  LimitOutput=off  UpperSaturationLimit=1  LowerSaturationLimit=0  LinearizeAsGain=off  AntiWindupMode=back-calculation  Kb=1  POutMin=[]  POutMax=[]  IOutMin=[]  IOutMax=[]  DOutMin=[]  DOutMax=[]  NOutMin=[]  NOutMax=[]  SumOutMin=[]  SumOutMax=[]  SaturationOutMin=[]  SaturationOutMax=[]  PParamMin=[]  PParamMax=[]  IParamMin=[]  IParamMax=[]  DParamMin=[]  DParamMax=[]  NParamMin=[]  NParamMax=[]  KbParamMin=[]  KbParamMax=[]  KtParamMin=[]  KtParamMax=[]  KbOutMin=[]  KbOutMax=[]  KtOutMin=[]  KtOutMax=[]  IntegratorOutMin=[]  IntegratorOutMax=[]  FilterOutMin=[]  FilterOutMax=[]  SumI1OutMin=[]  SumI1OutMax=[]  SumI2OutMin=[]  SumI2OutMax=[]  SumI3OutMin=[]  SumI3OutMax=[]  SumI4OutMin=[]  SumI4OutMax=[]  SumDOutMin=[]  SumDOutMax=[]  DifferentiatorOutMin=[]  DifferentiatorOutMax=[]  FilterDiffOutCoefMin=[]  FilterDiffOutCoefMax=[]  ReciprocalOutMin=[]  ReciprocalOutMax=[]  SumDenOutMin=[]  SumDenOutMax=[]  SumNumOutMin=[]  SumNumOutMax=[]  DivideOutMin=[]  DivideOutMax=[]  IntegratorContinuousStateAttributes=''  IntegratorStateMustResolveToSignalObject=off  IntegratorRTWStateStorageClass=Auto  FilterContinuousStateAttributes=''  FilterStateMustResolveToSignalObject=off  FilterRTWStateStorageClass=Auto  ParallelPVariant=InternalParameters  IdealPVariant=Disabled  IVariant=InternalParameters  DVariant=InternalParameters  IntegratorVariant=Discrete  SatVariant=Disabled  AWVariant=Passthrough  PCopyVariant=Disabled  TRVariant=Disabled  FdbkBlocksVariant=Forward  IdealPFdbkVariant=Disabled  SatFdbkVariant=Disabled  DerivativeFilterVariant=ForwardEulerFilter  NVariant=InternalParameters  NCopyVariant=Disabled  FilterICVariant=InternalICsFilter  IntegratorICVariant=InternalICs  ExternalResetVariant=Disabled  TRSumVariant=Passthrough  SumFdbkVariant=Disabled  SumVariant=Sum_PID
  PWM Generator (DC-DC) : powerlib_meascontrol/Pulse & Signal Generators/PWM Generator (DC-DC)  Fsw=10e3  Ts=0
      settings: SourceProductName=Simscape Electrical
  Saturation : Saturate  UpperLimit=1  LowerLimit=0
  Scope : Scope
  tag scope: G_BAT=global
  wires:
  Saturation/1 -> PWM Generator (DC-DC)/1
  Mux/1 -> [G_BAT]
  Constant/1 -> Add3/1
  Add3/1 -> PID Controller/1
  PID Controller1/1 -> Saturation/1
  NOT/1 -> Cast To Double/1
  PWM Generator (DC-DC)/1 -> Mux/2, NOT/1
  PID Controller/1 -> Gain/1, Scope/1  "Iload"
  Cast To Double/1 -> Mux/1
  Add1/1 -> PID Controller1/1
  [Vdc] -> Add3/2
  [Ibat] -> Add1/2
  Gain/1 -> Add1/1

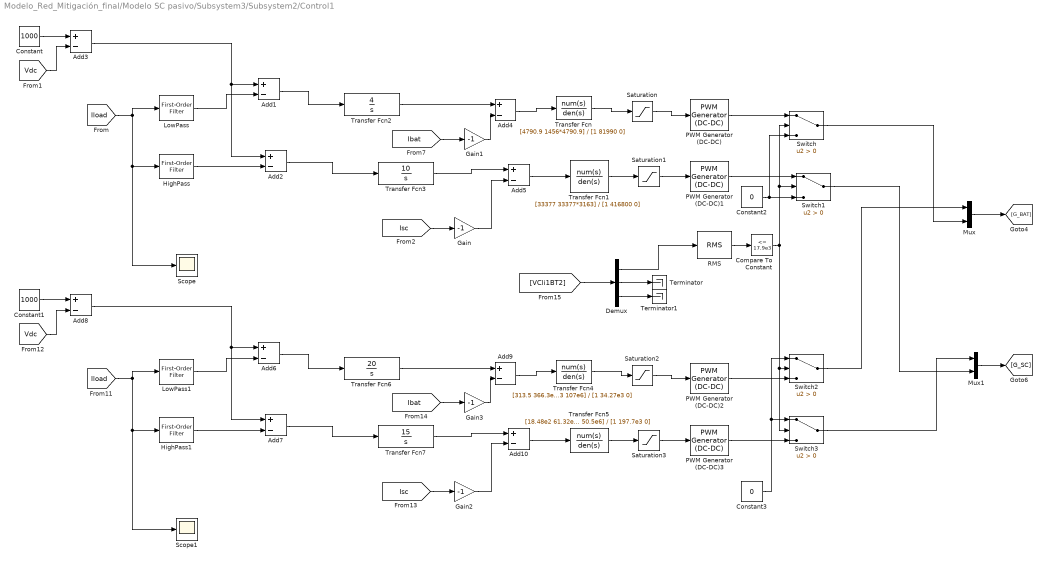
== system Modelo_Red_Mitigación_final/Modelo SC pasivo/Subsystem3/Subsystem2/Control1  ==
  Add{1..10} (10 alike) : Sum  Inputs=+-
  Compare To Constant : simulink/Logic and Bit Operations/Compare To Constant  relop=<=  const=17.9e3  OutDataTypeStr=boolean
  Constant : Constant  Value=1000
  Constant1 : Constant  Value=1000
  Constant2 : Constant  Value=0
  Constant3 : Constant  Value=0
  Demux : Demux  Outputs=3
  Gain{,1..3} (4 alike) : Gain  Gain=-1
  HighPass : powerlib_meascontrol/Filters/First-Order Filter  FilterType=Highpass  Tc=10e-3  Ts=0  Initialize=on  Vac_Init=[0, 0, 60]  Vdc_Init=0  PlotResponse=off  FreqRange="[0,  200,  1]"
      settings: SourceProductName=Simscape Electrical
  HighPass1 : powerlib_meascontrol/Filters/First-Order Filter  FilterType=Highpass  Tc=10e-3  Ts=0  Initialize=on  Vac_Init=[0, 0, 60]  Vdc_Init=0  PlotResponse=off  FreqRange="[0,  200,  1]"
      settings: SourceProductName=Simscape Electrical
  LowPass : powerlib_meascontrol/Filters/First-Order Filter  FilterType=Lowpass  Tc=10e-3  Ts=0  Initialize=on  Vac_Init=[0, 0, 60]  Vdc_Init=0  PlotResponse=off  FreqRange="[0,  200,  1]"
      settings: SourceProductName=Simscape Electrical
  LowPass1 : powerlib_meascontrol/Filters/First-Order Filter  FilterType=Lowpass  Tc=10e-3  Ts=0  Initialize=on  Vac_Init=[0, 0, 60]  Vdc_Init=0  PlotResponse=off  FreqRange="[0,  200,  1]"
      settings: SourceProductName=Simscape Electrical
  Mux : Mux  Inputs=2
  Mux1 : Mux  Inputs=2
  PWM Generator (DC-DC) : powerlib_meascontrol/Pulse & Signal Generators/PWM Generator (DC-DC)  Fsw=10e3  Ts=0
      settings: SourceProductName=Simscape Electrical
  PWM Generator (DC-DC)1 : powerlib_meascontrol/Pulse & Signal Generators/PWM Generator (DC-DC)  Fsw=30e3  Ts=0
      settings: SourceProductName=Simscape Electrical
  PWM Generator (DC-DC)2 : powerlib_meascontrol/Pulse & Signal Generators/PWM Generator (DC-DC)  Fsw=10e3  Ts=0
      settings: SourceProductName=Simscape Electrical
  PWM Generator (DC-DC)3 : powerlib_meascontrol/Pulse & Signal Generators/PWM Generator (DC-DC)  Fsw=30e3  Ts=0
      settings: SourceProductName=Simscape Electrical
  RMS : powerlib_meascontrol/Measurements/RMS  TrueRMS=on  Freq=60  RMSInit=19.9e3  Ts=0
      settings: SourceProductName=Simscape Electrical
  Saturation{,1..3} (4 alike) : Saturate  UpperLimit=1  LowerLimit=0
  Scope : Scope
  Scope1 : Scope
  Switch{,1..3} (4 alike) : Switch  Criteria=u2 > Threshold
  Terminator : Terminator
  Terminator1 : Terminator
  Transfer Fcn : TransferFcn  Numerator=[4790.9 1456*4790.9]  Denominator=[1 81990 0]
  Transfer Fcn1 : TransferFcn  Numerator=[33377 33377*3163]  Denominator=[1 416800 0]
  Transfer Fcn2 : TransferFcn  Numerator=[4]  Denominator=[1 0]
  Transfer Fcn3 : TransferFcn  Numerator=[10]  Denominator=[1 0]
  Transfer Fcn4 : TransferFcn  Numerator=[313.5 366.3e3 107e6]  Denominator=[1 34.27e3 0]
  Transfer Fcn5 : TransferFcn  Numerator=[18.48e2 61.32e3 50.5e6]  Denominator=[1 197.7e3 0]
  Transfer Fcn6 : TransferFcn  Numerator=[20]  Denominator=[1 0]
  Transfer Fcn7 : TransferFcn  Numerator=[15]  Denominator=[1 0]
  wires:
  Compare To Constant/1 -> Switch3/2, Switch2/2, Switch1/2, Switch/2
  Add10/1 -> Transfer Fcn5/1
  HighPass1/1 -> Add7/2
  Switch2/1 -> Mux/1
  Add3/1 -> Add2/1, Add1/1
  LowPass/1 -> Add1/2
  Demux/2 -> Terminator/1
  Add4/1 -> Transfer Fcn/1
  Constant2/1 -> Switch/3, Switch1/3
  Transfer Fcn2/1 -> Add4/1
  Add6/1 -> Transfer Fcn6/1
  Gain2/1 -> Add10/2
  Saturation/1 -> PWM Generator (DC-DC)/1
  Gain3/1 -> Add9/2
  Constant1/1 -> Add8/1
  Demux/3 -> Terminator1/1
  Transfer Fcn7/1 -> Add10/1
  Switch1/1 -> Mux1/2
  Add9/1 -> Transfer Fcn4/1
  Transfer Fcn6/1 -> Add9/1
  Transfer Fcn5/1 -> Saturation3/1
  Saturation1/1 -> PWM Generator (DC-DC)1/1
  Transfer Fcn4/1 -> Saturation2/1
  Mux1/1 -> [G_SC]
  [Iload] -> Scope1/1, HighPass1/1, LowPass1/1
  [Isc] -> Gain2/1
  Saturation3/1 -> PWM Generator (DC-DC)3/1
  HighPass/1 -> Add2/2
  [Ibat] -> Gain3/1
  [Vdc] -> Add8/2
  Gain/1 -> Add5/2
  [Isc] -> Gain/1
  Saturation2/1 -> PWM Generator (DC-DC)2/1
  PWM Generator (DC-DC)3/1 -> Switch3/3
  Add8/1 -> Add7/1, Add6/1
  Add7/1 -> Transfer Fcn7/1
  Transfer Fcn1/1 -> Saturation1/1
  Switch3/1 -> Mux1/1
  Gain1/1 -> Add4/2
  Constant3/1 -> Switch2/1, Switch3/1
  LowPass1/1 -> Add6/2
  RMS/1 -> Compare To Constant/1
  PWM Generator (DC-DC)1/1 -> Switch1/1
  Transfer Fcn3/1 -> Add5/1
  Add2/1 -> Transfer Fcn3/1
  Demux/1 -> RMS/1
  PWM Generator (DC-DC)/1 -> Switch/1
  Transfer Fcn/1 -> Saturation/1
  PWM Generator (DC-DC)2/1 -> Switch2/3
  Switch/1 -> Mux/2
  [Iload] -> Scope/1, HighPass/1, LowPass/1
  [Ibat] -> Gain1/1
  Mux/1 -> [G_BAT]
  Add1/1 -> Transfer Fcn2/1
  Add5/1 -> Transfer Fcn1/1
  [Vdc] -> Add3/2
  [VCli1BT2] -> Demux/1
  Constant/1 -> Add3/1

== system Modelo_Red_Mitigación_final/Modelo SC pasivo/Subsystem3/Subsystem2/Control2 ==
  Add : Sum
  Add1 : Sum  Inputs=+-
  Add2 : Sum  Inputs=+-
  Add3 : Sum  Inputs=+-
  Cast To Double : DataTypeConversion  OutDataTypeStr=double
  Cast To Double1 : DataTypeConversion  OutDataTypeStr=double
  Constant : Constant  Value=1000
  Gain : Gain  Gain=-1
  Gain1 : Gain  Gain=-1
  HighPass : powerlib_meascontrol/Filters/First-Order Filter  FilterType=Highpass  Tc=10e-3  Ts=0  Initialize=on  Vac_Init=[0, 0, 60]  Vdc_Init=0  PlotResponse=off  FreqRange="[0,  200,  1]"
      settings: SourceProductName=Simscape Electrical
  LowPass : powerlib_meascontrol/Filters/First-Order Filter  FilterType=Lowpass  Tc=10e-3  Ts=0  Initialize=on  Vac_Init=[0, 0, 60]  Vdc_Init=0  PlotResponse=off  FreqRange="[0,  200,  1]"
      settings: SourceProductName=Simscape Electrical
  Mux : Mux  Inputs=2
  Mux1 : Mux  Inputs=2
  NOT : Logic  Operator=NOT  IconShape=distinctive  AllPortsSameDT=off  OutDataTypeStr=boolean
  NOT1 : Logic  Operator=NOT  IconShape=distinctive  AllPortsSameDT=off  OutDataTypeStr=boolean
  PID Controller : simulink/Continuous/PID Controller  Controller=PID  Form=Parallel  TimeDomain=Continuous-time  SampleTime=-1  IntegratorMethod=Forward Euler  FilterMethod=Forward Euler  ControllerParametersSource=internal  P=5  I=1  D=0  UseFilter=on  N=100  TunerSelectOption=Transfer Function Based (PID Tuner App)  InitialConditionSource=internal  InitialConditionForIntegrator=0  InitialConditionForFilter=0  DifferentiatorICPrevScaledInput=0  ExternalReset=none  TrackingMode=off  Kt=1  LimitOutput=off  UpperSaturationLimit=inf  LowerSaturationLimit=-inf  LinearizeAsGain=on  AntiWindupMode=none  Kb=1  POutMin=[]  POutMax=[]  IOutMin=[]  IOutMax=[]  DOutMin=[]  DOutMax=[]  NOutMin=[]  NOutMax=[]  SumOutMin=[]  SumOutMax=[]  SaturationOutMin=[]  SaturationOutMax=[]  PParamMin=[]  PParamMax=[]  IParamMin=[]  IParamMax=[]  DParamMin=[]  DParamMax=[]  NParamMin=[]  NParamMax=[]  KbParamMin=[]  KbParamMax=[]  KtParamMin=[]  KtParamMax=[]  KbOutMin=[]  KbOutMax=[]  KtOutMin=[]  KtOutMax=[]  IntegratorOutMin=[]  IntegratorOutMax=[]  FilterOutMin=[]  FilterOutMax=[]  SumI1OutMin=[]  SumI1OutMax=[]  SumI2OutMin=[]  SumI2OutMax=[]  SumI3OutMin=[]  SumI3OutMax=[]  SumI4OutMin=[]  SumI4OutMax=[]  SumDOutMin=[]  SumDOutMax=[]  DifferentiatorOutMin=[]  DifferentiatorOutMax=[]  FilterDiffOutCoefMin=[]  FilterDiffOutCoefMax=[]  ReciprocalOutMin=[]  ReciprocalOutMax=[]  SumDenOutMin=[]  SumDenOutMax=[]  SumNumOutMin=[]  SumNumOutMax=[]  DivideOutMin=[]  DivideOutMax=[]  IntegratorContinuousStateAttributes=''  IntegratorStateMustResolveToSignalObject=off  IntegratorRTWStateStorageClass=Auto  FilterContinuousStateAttributes=''  FilterStateMustResolveToSignalObject=off  FilterRTWStateStorageClass=Auto  ParallelPVariant=InternalParameters  IdealPVariant=Disabled  IVariant=InternalParameters  DVariant=InternalParameters  IntegratorVariant=Continuous  SatVariant=Disabled  AWVariant=Passthrough  PCopyVariant=Disabled  TRVariant=Disabled  FdbkBlocksVariant=Forward  IdealPFdbkVariant=Disabled  SatFdbkVariant=Disabled  DerivativeFilterVariant=ContFilter  NVariant=InternalParameters  NCopyVariant=Disabled  FilterICVariant=InternalICsFilter  IntegratorICVariant=InternalICs  ExternalResetVariant=Disabled  TRSumVariant=Passthrough  SumFdbkVariant=Disabled  SumVariant=Sum_PID
  PID Controller1 : simulink/Continuous/PID Controller  Controller=PID  Form=Parallel  TimeDomain=Continuous-time  SampleTime=-1  IntegratorMethod=Forward Euler  FilterMethod=Forward Euler  ControllerParametersSource=internal  P=10  I=2  D=0  UseFilter=on  N=100  TunerSelectOption=Transfer Function Based (PID Tuner App)  InitialConditionSource=internal  InitialConditionForIntegrator=0  InitialConditionForFilter=0  DifferentiatorICPrevScaledInput=0  ExternalReset=none  TrackingMode=off  Kt=1  LimitOutput=off  UpperSaturationLimit=inf  LowerSaturationLimit=-inf  LinearizeAsGain=on  AntiWindupMode=none  Kb=1  POutMin=[]  POutMax=[]  IOutMin=[]  IOutMax=[]  DOutMin=[]  DOutMax=[]  NOutMin=[]  NOutMax=[]  SumOutMin=[]  SumOutMax=[]  SaturationOutMin=[]  SaturationOutMax=[]  PParamMin=[]  PParamMax=[]  IParamMin=[]  IParamMax=[]  DParamMin=[]  DParamMax=[]  NParamMin=[]  NParamMax=[]  KbParamMin=[]  KbParamMax=[]  KtParamMin=[]  KtParamMax=[]  KbOutMin=[]  KbOutMax=[]  KtOutMin=[]  KtOutMax=[]  IntegratorOutMin=[]  IntegratorOutMax=[]  FilterOutMin=[]  FilterOutMax=[]  SumI1OutMin=[]  SumI1OutMax=[]  SumI2OutMin=[]  SumI2OutMax=[]  SumI3OutMin=[]  SumI3OutMax=[]  SumI4OutMin=[]  SumI4OutMax=[]  SumDOutMin=[]  SumDOutMax=[]  DifferentiatorOutMin=[]  DifferentiatorOutMax=[]  FilterDiffOutCoefMin=[]  FilterDiffOutCoefMax=[]  ReciprocalOutMin=[]  ReciprocalOutMax=[]  SumDenOutMin=[]  SumDenOutMax=[]  SumNumOutMin=[]  SumNumOutMax=[]  DivideOutMin=[]  DivideOutMax=[]  IntegratorContinuousStateAttributes=''  IntegratorStateMustResolveToSignalObject=off  IntegratorRTWStateStorageClass=Auto  FilterContinuousStateAttributes=''  FilterStateMustResolveToSignalObject=off  FilterRTWStateStorageClass=Auto  ParallelPVariant=InternalParameters  IdealPVariant=Disabled  IVariant=InternalParameters  DVariant=InternalParameters  IntegratorVariant=Continuous  SatVariant=Disabled  AWVariant=Passthrough  PCopyVariant=Disabled  TRVariant=Disabled  FdbkBlocksVariant=Forward  IdealPFdbkVariant=Disabled  SatFdbkVariant=Disabled  DerivativeFilterVariant=ContFilter  NVariant=InternalParameters  NCopyVariant=Disabled  FilterICVariant=InternalICsFilter  IntegratorICVariant=InternalICs  ExternalResetVariant=Disabled  TRSumVariant=Passthrough  SumFdbkVariant=Disabled  SumVariant=Sum_PID
  PID Controller2 : simulink/Continuous/PID Controller  Controller=PID  Form=Parallel  TimeDomain=Continuous-time  SampleTime=-1  IntegratorMethod=Forward Euler  FilterMethod=Forward Euler  ControllerParametersSource=internal  P=50  I=10  D=0  UseFilter=on  N=100  TunerSelectOption=Transfer Function Based (PID Tuner App)  InitialConditionSource=internal  InitialConditionForIntegrator=0  InitialConditionForFilter=0  DifferentiatorICPrevScaledInput=0  ExternalReset=none  TrackingMode=off  Kt=1  LimitOutput=off  UpperSaturationLimit=inf  LowerSaturationLimit=-inf  LinearizeAsGain=on  AntiWindupMode=none  Kb=1  POutMin=[]  POutMax=[]  IOutMin=[]  IOutMax=[]  DOutMin=[]  DOutMax=[]  NOutMin=[]  NOutMax=[]  SumOutMin=[]  SumOutMax=[]  SaturationOutMin=[]  SaturationOutMax=[]  PParamMin=[]  PParamMax=[]  IParamMin=[]  IParamMax=[]  DParamMin=[]  DParamMax=[]  NParamMin=[]  NParamMax=[]  KbParamMin=[]  KbParamMax=[]  KtParamMin=[]  KtParamMax=[]  KbOutMin=[]  KbOutMax=[]  KtOutMin=[]  KtOutMax=[]  IntegratorOutMin=[]  IntegratorOutMax=[]  FilterOutMin=[]  FilterOutMax=[]  SumI1OutMin=[]  SumI1OutMax=[]  SumI2OutMin=[]  SumI2OutMax=[]  SumI3OutMin=[]  SumI3OutMax=[]  SumI4OutMin=[]  SumI4OutMax=[]  SumDOutMin=[]  SumDOutMax=[]  DifferentiatorOutMin=[]  DifferentiatorOutMax=[]  FilterDiffOutCoefMin=[]  FilterDiffOutCoefMax=[]  ReciprocalOutMin=[]  ReciprocalOutMax=[]  SumDenOutMin=[]  SumDenOutMax=[]  SumNumOutMin=[]  SumNumOutMax=[]  DivideOutMin=[]  DivideOutMax=[]  IntegratorContinuousStateAttributes=''  IntegratorStateMustResolveToSignalObject=off  IntegratorRTWStateStorageClass=Auto  FilterContinuousStateAttributes=''  FilterStateMustResolveToSignalObject=off  FilterRTWStateStorageClass=Auto  ParallelPVariant=InternalParameters  IdealPVariant=Disabled  IVariant=InternalParameters  DVariant=InternalParameters  IntegratorVariant=Continuous  SatVariant=Disabled  AWVariant=Passthrough  PCopyVariant=Disabled  TRVariant=Disabled  FdbkBlocksVariant=Forward  IdealPFdbkVariant=Disabled  SatFdbkVariant=Disabled  DerivativeFilterVariant=ContFilter  NVariant=InternalParameters  NCopyVariant=Disabled  FilterICVariant=InternalICsFilter  IntegratorICVariant=InternalICs  ExternalResetVariant=Disabled  TRSumVariant=Passthrough  SumFdbkVariant=Disabled  SumVariant=Sum_PID
  PWM Generator (DC-DC) : powerlib_meascontrol/Pulse & Signal Generators/PWM Generator (DC-DC)  Fsw=10e3  Ts=0
      settings: SourceProductName=Simscape Electrical
  PWM Generator (DC-DC)1 : powerlib_meascontrol/Pulse & Signal Generators/PWM Generator (DC-DC)  Fsw=30e3  Ts=0
      settings: SourceProductName=Simscape Electrical
  Saturation : Saturate  UpperLimit=1  LowerLimit=0
  Saturation1 : Saturate  UpperLimit=1  LowerLimit=0
  Scope : Scope
  tag scope: G_BAT=global, G_SC=global
  wires:
  Saturation/1 -> PWM Generator (DC-DC)/1
  Saturation1/1 -> PWM Generator (DC-DC)1/1
  Mux1/1 -> [G_SC]
  [Isc] -> Gain/1
  PID Controller2/1 -> Saturation1/1
  [Iload] -> Scope/1, HighPass/1, LowPass/1
  [Ibat] -> Gain1/1
  Mux/1 -> [G_BAT]
  [Vdc] -> Add3/2
  Constant/1 -> Add3/1
  Add3/1 -> PID Controller/1
  PID Controller/1 -> Add/1
  LowPass/1 -> Add/2
  Add/1 -> Add1/1
  Gain1/1 -> Add1/2
  Add1/1 -> PID Controller1/1
  PID Controller1/1 -> Saturation/1
  Gain/1 -> Add2/2
  HighPass/1 -> Add2/1
  Add2/1 -> PID Controller2/1
  NOT/1 -> Cast To Double/1
  Cast To Double/1 -> Mux/1
  PWM Generator (DC-DC)/1 -> Mux/2, NOT/1
  NOT1/1 -> Cast To Double1/1
  PWM Generator (DC-DC)1/1 -> Mux1/2, NOT1/1
  Cast To Double1/1 -> Mux1/1

== system Modelo_Red_Mitigación_final/Modelo bateria pasiva/Subsystem2/Subsystem/Subsystem ==
  In1 : Inport
  Cast To Boolean : DataTypeConversion  OutDataTypeStr=boolean
  Cast To Boolean1 : DataTypeConversion  OutDataTypeStr=boolean
  Cast To Double : DataTypeConversion  OutDataTypeStr=double
  Clock : simulink_extras/Flip Flops/Clock  period=1/10e3
  Constant1 : Constant  Value=0
  Constant2 : Constant
  Constant3 : Constant  Value=0
  Mux : Mux  Inputs=2
  S-R Flip-Flop : simulink_extras/Flip Flops/S-R Flip-Flop  initial_condition=1
  Switch : Switch  Criteria=u2 > Threshold
  Out1 : Outport
  Out2 : Outport  Port=2
  wires:
  S-R Flip-Flop/2 -> Out2/1
  In1/1 -> Switch/2
  Clock/1 -> Cast To Boolean/1
  Mux/1 -> Out1/1
  Cast To Boolean1/1 -> S-R Flip-Flop/2
  Switch/1 -> Cast To Boolean1/1
  Constant3/1 -> Switch/3
  Constant1/1 -> Mux/1
  Cast To Boolean/1 -> S-R Flip-Flop/1
  Cast To Double/1 -> Mux/2
  Constant2/1 -> Switch/1
  S-R Flip-Flop/1 -> Cast To Double/1
